simulink model "chap04"  (R2021a)
settings: Solver=FixedStepDiscrete  StartTime=0.0  StopTime=30  FixedStep=0.001  RelTol=1e-3
undefined symbols (not defined in the file): DiscIntNeverNeededParam
libraries: simulink x4
(part 7 of 7)

== matlab function chap04/Subsystem/Subsystem/Subsystem12/MATLAB Function ==
  data: u input; y output
function y = fcn(u)

y = norm(u);

== matlab function chap04/Subsystem/Subsystem/Subsystem12/MATLAB Function3 ==
  data: u input; y output
function y = fcn(u)

y = norm(u);

== matlab function chap04/Subsystem/Subsystem2/Subsystem12/MATLAB Function3 ==
  data: u input; y output
function y = fcn(u)

y = norm(u);

== matlab function chap04/Subsystem/Subsystem/Subsystem4/Subsystem/MATLAB Function ==
  data: u1 input; y output; u2 input
function y = fcn(u1,u2)


if (u1==u2)
    y = 0;
else
    y = 1;
end

== matlab function chap04/Subsystem/Subsystem5/Subsystem12/MATLAB Function ==
  data: u input; y output
function y = fcn(u)

y = norm(u);

== matlab function chap04/Subsystem/Subsystem5/Subsystem4/Subsystem/MATLAB Function ==
  data: u1 input; y output; u2 input
function y = fcn(u1,u2)


if (u1==u2)
    y = 0;
else
    y = 1;
end

== matlab function chap04/Subsystem/Subsystem5/Subsystem7/Subsystem/MATLAB Function ==
  data: u1 input; y output; u2 input
function y = fcn(u1,u2)


if (u1==u2)
    y = 0;
else
    y = 1;
end

== matlab function chap04/Subsystem/Subsystem6/MATLAB Function ==
  data: u input; y output
function y = fcn(u)

y = norm(u);

== matlab function chap04/Subsystem/Subsystem5/Subsystem8/Subsystem/MATLAB Function ==
  data: u1 input; y output; u2 input
function y = fcn(u1,u2)


if (u1==u2)
    y = 0;
else
    y = 1;
end

== matlab function chap04/Subsystem/Subsystem5/Subsystem12/MATLAB Function3 ==
  data: u input; y output
function y = fcn(u)

y = norm(u);

== matlab function chap04/Subsystem/Subsystem3/Subsystem12/MATLAB Function ==
  data: u input; y output
function y = fcn(u)

y = norm(u);

== matlab function chap04/Subsystem/Subsystem3/Subsystem12/MATLAB Function3 ==
  data: u input; y output
function y = fcn(u)

y = norm(u);

== matlab function chap04/Subsystem/Subsystem3/Subsystem4/Subsystem/MATLAB Function ==
  data: u1 input; y output; u2 input
function y = fcn(u1,u2)


if (u1==u2)
    y = 0;
else
    y = 1;
end

== matlab function chap04/Subsystem/Subsystem3/Subsystem7/Subsystem/MATLAB Function ==
  data: u1 input; y output; u2 input
function y = fcn(u1,u2)


if (u1==u2)
    y = 0;
else
    y = 1;
end

== matlab function chap04/Subsystem/Subsystem4/Subsystem4/Subsystem/MATLAB Function ==
  data: u1 input; y output; u2 input
function y = fcn(u1,u2)


if (u1==u2)
    y = 0;
else
    y = 1;
end

== matlab function chap04/Subsystem/Subsystem4/Subsystem7/Subsystem/MATLAB Function ==
  data: u1 input; y output; u2 input
function y = fcn(u1,u2)


if (u1==u2)
    y = 0;
else
    y = 1;
end

== matlab function chap04/Subsystem/Subsystem4/Subsystem8/Subsystem/MATLAB Function ==
  data: u1 input; y output; u2 input
function y = fcn(u1,u2)


if (u1==u2)
    y = 0;
else
    y = 1;
end

== matlab function chap04/Subsystem/Subsystem6/MATLAB Function2 ==
  data: u input; y output
function y = fcn(u)

y = norm(u);

== matlab function chap04/Subsystem/Subsystem3/Subsystem8/Subsystem/MATLAB Function ==
  data: u1 input; y output; u2 input
function y = fcn(u1,u2)


if (u1==u2)
    y = 0;
else
    y = 1;
end

== matlab function chap04/Subsystem/Subsystem1/Subsystem12/MATLAB Function ==
  data: u input; y output
function y = fcn(u)

y = norm(u);

== matlab function chap04/Subsystem/Subsystem1/Subsystem12/MATLAB Function3 ==
  data: u input; y output
function y = fcn(u)

y = norm(u);

== matlab function chap04/Subsystem/Subsystem4/Subsystem12/MATLAB Function ==
  data: u input; y output
function y = fcn(u)

y = norm(u);

== matlab function chap04/Subsystem/Subsystem4/Subsystem12/MATLAB Function3 ==
  data: u input; y output
function y = fcn(u)

y = norm(u);

== matlab function chap04/Subsystem/Subsystem2/Subsystem3/Subsystem2/MATLAB Function ==
  data: u input; y output
function y = fcn(u)

y = norm(u);

== matlab function chap04/Subsystem/Subsystem5/Subsystem3/Subsystem2/MATLAB Function ==
  data: u input; y output
function y = fcn(u)

y = norm(u);

== matlab function chap04/Subsystem/Subsystem3/Subsystem3/Subsystem2/MATLAB Function ==
  data: u input; y output
function y = fcn(u)

y = norm(u);

== matlab function chap04/Subsystem/Subsystem1/Subsystem3/Subsystem2/MATLAB Function ==
  data: u input; y output
function y = fcn(u)

y = norm(u);

== matlab function chap04/Subsystem/Subsystem4/Subsystem3/Subsystem2/MATLAB Function ==
  data: u input; y output
function y = fcn(u)

y = norm(u);

== matlab function chap04/Subsystem/Subsystem2/Subsystem7/Subsystem/MATLAB Function ==
  data: u1 input; y output; u2 input
function y = fcn(u1,u2)


if (u1==u2)
    y = 0;
else
    y = 1;
end

== matlab function chap04/Subsystem/Subsystem/Subsystem10/MATLAB Function ==
  data: u input; utk input; nrom output
function nrom = fcn(u,utk)

e = utk-u;
nrom = norm(e);

== matlab function chap04/Subsystem/Subsystem2/Subsystem10/MATLAB Function ==
  data: u input; utk input; nrom output
function nrom = fcn(u,utk)

e = utk-u;
nrom = norm(e);

== matlab function chap04/Subsystem/Subsystem5/Subsystem10/MATLAB Function ==
  data: u input; utk input; nrom output
function nrom = fcn(u,utk)

e = utk-u;
nrom = norm(e);

== matlab function chap04/Subsystem/Subsystem3/Subsystem10/MATLAB Function ==
  data: u input; utk input; nrom output
function nrom = fcn(u,utk)

e = utk-u;
nrom = norm(e);

== matlab function chap04/Subsystem/Subsystem1/Subsystem10/MATLAB Function ==
  data: u input; utk input; nrom output
function nrom = fcn(u,utk)

e = utk-u;
nrom = norm(e);

== matlab function chap04/Subsystem/Subsystem4/Subsystem10/MATLAB Function ==
  data: u input; utk input; nrom output
function nrom = fcn(u,utk)

e = utk-u;
nrom = norm(e);

== matlab function chap04/Subsystem/Subsystem/Subsystem3/MATLAB Function ==
  data: u input; y output
function y = fcn(u)

y = u;

if y==0
    y=10e-15;
end

== matlab function chap04/Subsystem/Subsystem/Subsystem3/MATLAB Function1 ==
  data: u input; y output
function y = fcn(u)

y = u;

if y==0
    y=10e-15;
end

== matlab function chap04/Subsystem/Subsystem/Subsystem3/MATLAB Function2 ==
  data: u input; y output
function y = fcn(u)

y = u;

if y==0
    y=10e-15;
end

== matlab function chap04/Subsystem/Subsystem/Subsystem3/Subsystem/MATLAB Function ==
  data: u input; y output
function y = fcn(u)

y = norm(u);

== matlab function chap04/Subsystem/Subsystem/Subsystem3/Subsystem1/MATLAB Function ==
  data: u input; y output
function y = fcn(u)

y = norm(u)^(1/2);

== matlab function chap04/Subsystem/Subsystem6/MATLAB Function3 ==
  data: u input; y output
function y = fcn(u)

y = norm(u);

== matlab function chap04/Subsystem/Subsystem/Subsystem3/Subsystem2/MATLAB Function ==
  data: u input; y output
function y = fcn(u)

y = norm(u);

== matlab function chap04/Subsystem/Subsystem2/Subsystem3/MATLAB Function ==
  data: u input; y output
function y = fcn(u)

y = u;

if y==0
    y=10e-15;
end

== matlab function chap04/Subsystem/Subsystem2/Subsystem3/MATLAB Function1 ==
  data: u input; y output
function y = fcn(u)

y = u;

if y==0
    y=10e-15;
end

== matlab function chap04/Subsystem/Subsystem2/Subsystem3/MATLAB Function2 ==
  data: u input; y output
function y = fcn(u)

y = u;

if y==0
    y=10e-15;
end

== matlab function chap04/Subsystem/Subsystem2/Subsystem3/Subsystem/MATLAB Function ==
  data: u input; y output
function y = fcn(u)

y = norm(u);

== matlab function chap04/Subsystem/Subsystem2/Subsystem3/Subsystem1/MATLAB Function ==
  data: u input; y output
function y = fcn(u)

y = norm(u)^(1/2);

== matlab function chap04/Subsystem/Subsystem5/Subsystem3/MATLAB Function ==
  data: u input; y output
function y = fcn(u)

y = u;

if y==0
    y=10e-15;
end

== matlab function chap04/Subsystem/Subsystem5/Subsystem3/MATLAB Function1 ==
  data: u input; y output
function y = fcn(u)

y = u;

if y==0
    y=10e-15;
end

== matlab function chap04/Subsystem/Subsystem5/Subsystem3/MATLAB Function2 ==
  data: u input; y output
function y = fcn(u)

y = u;

if y==0
    y=10e-15;
end

== matlab function chap04/Subsystem/Subsystem5/Subsystem3/Subsystem/MATLAB Function ==
  data: u input; y output
function y = fcn(u)

y = norm(u);

== matlab function chap04/Subsystem/Subsystem2/Subsystem8/Subsystem/MATLAB Function ==
  data: u1 input; y output; u2 input
function y = fcn(u1,u2)


if (u1==u2)
    y = 0;
else
    y = 1;
end

== matlab function chap04/Subsystem/Subsystem5/Subsystem3/Subsystem1/MATLAB Function ==
  data: u input; y output
function y = fcn(u)

y = norm(u)^(1/2);

== matlab function chap04/Subsystem/Subsystem3/Subsystem3/MATLAB Function ==
  data: u input; y output
function y = fcn(u)

y = u;

if y==0
    y=10e-15;
end

== matlab function chap04/Subsystem/Subsystem3/Subsystem3/MATLAB Function1 ==
  data: u input; y output
function y = fcn(u)

y = u;

if y==0
    y=10e-15;
end

== matlab function chap04/Subsystem/Subsystem3/Subsystem3/MATLAB Function2 ==
  data: u input; y output
function y = fcn(u)

y = u;

if y==0
    y=10e-15;
end

== matlab function chap04/Subsystem/Subsystem3/Subsystem3/Subsystem/MATLAB Function ==
  data: u input; y output
function y = fcn(u)

y = norm(u);

== matlab function chap04/Subsystem/Subsystem3/Subsystem3/Subsystem1/MATLAB Function ==
  data: u input; y output
function y = fcn(u)

y = norm(u)^(1/2);

== matlab function chap04/Subsystem/Subsystem1/Subsystem3/MATLAB Function ==
  data: u input; y output
function y = fcn(u)

y = u;

if y==0
    y=10e-15;
end

== matlab function chap04/Subsystem/Subsystem1/Subsystem3/MATLAB Function1 ==
  data: u input; y output
function y = fcn(u)

y = u;

if y==0
    y=10e-15;
end

== matlab function chap04/Subsystem/Subsystem1/Subsystem3/MATLAB Function2 ==
  data: u input; y output
function y = fcn(u)

y = u;

if y==0
    y=10e-15;
end

== matlab function chap04/Subsystem/Subsystem1/Subsystem3/Subsystem/MATLAB Function ==
  data: u input; y output
function y = fcn(u)

y = norm(u);

== matlab function chap04/Subsystem/Subsystem1/Subsystem3/Subsystem1/MATLAB Function ==
  data: u input; y output
function y = fcn(u)

y = norm(u)^(1/2);

== matlab function chap04/Subsystem/Subsystem1/Subsystem4/Subsystem/MATLAB Function ==
  data: u1 input; y output; u2 input
function y = fcn(u1,u2)


if (u1==u2)
    y = 0;
else
    y = 1;
end

== matlab function chap04/Subsystem/Subsystem4/Subsystem3/MATLAB Function ==
  data: u input; y output
function y = fcn(u)

y = u;

if y==0
    y=10e-15;
end

== matlab function chap04/Subsystem/Subsystem4/Subsystem3/MATLAB Function1 ==
  data: u input; y output
function y = fcn(u)

y = u;

if y==0
    y=10e-15;
end

== matlab function chap04/Subsystem/Subsystem4/Subsystem3/MATLAB Function2 ==
  data: u input; y output
function y = fcn(u)

y = u;

if y==0
    y=10e-15;
end

== matlab function chap04/Subsystem/Subsystem4/Subsystem3/Subsystem/MATLAB Function ==
  data: u input; y output
function y = fcn(u)

y = norm(u);

== matlab function chap04/Subsystem/Subsystem4/Subsystem3/Subsystem1/MATLAB Function ==
  data: u input; y output
function y = fcn(u)

y = norm(u)^(1/2);

== matlab function chap04/Subsystem/Subsystem13/MATLAB Function ==
  data: u input; y output
function y = fcn(u)

y = norm(u);

== matlab function chap04/Subsystem/Subsystem13/MATLAB Function2 ==
  data: u input; y output
function y = fcn(u)

y = norm(u);

== matlab function chap04/Subsystem/Subsystem13/MATLAB Function3 ==
  data: u input; y output
function y = fcn(u)

y = norm(u);

== matlab function chap04/Subsystem/Subsystem9/MATLAB Function ==
  data: u input; y output
function y = fcn(u)

y = norm(u);

== matlab function chap04/Subsystem/Subsystem9/MATLAB Function2 ==
  data: u input; y output
function y = fcn(u)

y = norm(u);

== matlab function chap04/Subsystem/Subsystem9/MATLAB Function3 ==
  data: u input; y output
function y = fcn(u)

y = norm(u);

== matlab function chap04/Subsystem/Subsystem1/Subsystem7/Subsystem/MATLAB Function ==
  data: u1 input; y output; u2 input
function y = fcn(u1,u2)


if (u1==u2)
    y = 0;
else
    y = 1;
end

== matlab function chap04/Subsystem/Subsystem1/Subsystem8/Subsystem/MATLAB Function ==
  data: u1 input; y output; u2 input
function y = fcn(u1,u2)


if (u1==u2)
    y = 0;
else
    y = 1;
end

== matlab function chap04/Subsystem/Subsystem10/MATLAB Function ==
  data: u input; y output
function y = fcn(u)

y = norm(u);

== matlab function chap04/Subsystem/Subsystem10/MATLAB Function2 ==
  data: u input; y output
function y = fcn(u)

y = norm(u);

== matlab function chap04/Subsystem/Subsystem10/MATLAB Function3 ==
  data: u input; y output
function y = fcn(u)

y = norm(u);
